simulink model "mpptmodel_newtest"  (Simulink 10.0)
settings: Solver=ode45  StartTime=0.0  StopTime=20  FixedStep=1e-8  RelTol=1e-3  EnableMultiTasking=on
libraries: powerlib x13, simulink x3
settings Model: Creator=Ranjith  LastModifiedBy=bhisma
settings DataIOCC: LimitDataPoints=on  SignalLoggingSaveFormat=ModelDataLogs
settings OptimizationCC: ExpressionDepthLimit=2147483647
settings DebuggingCC: SolverPrmCheckMsg=warning  MultiTaskRateTransMsg=warning  FcnCallInpInsideContextMsg=warning  StateNameClashWarn=warning
settings GRTTargetCC: GeneratePreprocessorConditionals=Disable all  CombineOutputUpdateFcns=on  GRTInterface=off
settings ConfigComp: CovExternalEMLEnable=off
settings SimscapeCC: SimscapeNormalizeSystem=off

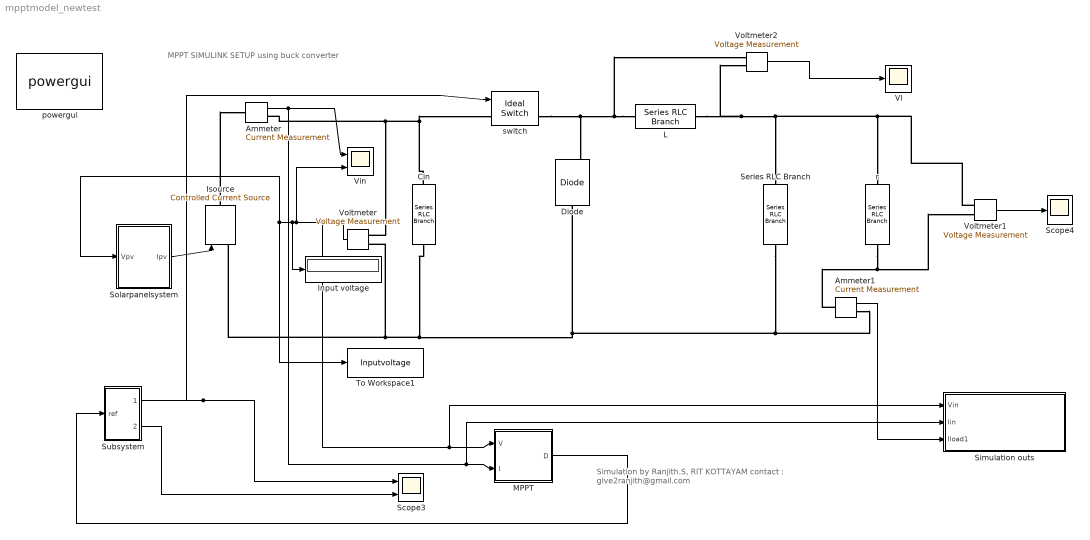
== system mpptmodel_newtest ==
  note: MPPT SIMULINK SETUP using buck converter
  note: Simulation by Ranjith.S, RIT KOTTAYAM
      |                          contact : give2ranjith@gmail.com
  Ammeter : powerlib/Measurements/Current Measurement  PhasorSimulation=off  OutputType=Complex  PSBequivalent=0
      settings: SourceProductName=Simscape Electrical
  Ammeter1 : powerlib/Measurements/Current Measurement  PhasorSimulation=off  OutputType=Complex  PSBequivalent=0
      settings: SourceProductName=Simscape Electrical
  Cin : powerlib/Elements/Series RLC Branch  LConnTagsString=__new0  RConnTagsString=__new0  BranchType=C  Resistance=0.03  Inductance=1e-3  SetiL0=off  InitialCurrent=0  Capacitance=2000e-6  Setx0=off  InitialVoltage=0  Measurements=None
      settings: SourceProductName=Simscape Electrical
  Diode : powerlib/Power Electronics/Diode  Ron=0.001  Lon=0  Vf=0.8  IC=0  UseSnubber=off  Rs=500  Cs=250e-9  Measurements=on
      settings: SourceProductName=Simscape Electrical
  Input voltage : Display
  Isource : powerlib/Electrical Sources/Controlled Current Source  Initialize=on  Source_Type=AC  Amplitude=0  Phase=0  Frequency=0  Measurements=None
      settings: SourceProductName=Simscape Electrical
  L : powerlib/Elements/Series RLC Branch  LConnTagsString=__new0  RConnTagsString=__new0  BranchType=L  Resistance=0.2e-3  Inductance=66e-6  SetiL0=off  InitialCurrent=0  Capacitance=1e-6  Setx0=off  InitialVoltage=0  Measurements=None
      settings: SourceProductName=Simscape Electrical
  MPPT : Subsystem
  Scope3 : Scope  NumInputPorts=2
  Scope4 : Scope
  Series RLC Branch : powerlib/Elements/Series RLC Branch  LConnTagsString=__new0  RConnTagsString=__new0  BranchType=RC  Resistance=0.0003  Inductance=1e-3  SetiL0=off  InitialCurrent=0  Capacitance=75e-6  Setx0=off  InitialVoltage=0  Measurements=None
      settings: SourceProductName=Simscape Electrical
  Simulation outs : Subsystem
  Solarpanelsystem : Subsystem
  Subsystem : Subsystem
  To Workspace1 : ToWorkspace  VariableName=Inputvoltage  SaveFormat=Timeseries  SampleTime=-1
  Vin : Scope  NumInputPorts=2
  Vl : Scope
  Voltmeter : powerlib/Measurements/Voltage Measurement  PhasorSimulation=off  OutputType=Complex  PSBequivalent=0
      settings: SourceProductName=Simscape Electrical
  Voltmeter1 : powerlib/Measurements/Voltage Measurement  PhasorSimulation=off  OutputType=Complex  PSBequivalent=0
      settings: SourceProductName=Simscape Electrical
  Voltmeter2 : powerlib/Measurements/Voltage Measurement  PhasorSimulation=off  OutputType=Complex  PSBequivalent=0
      settings: SourceProductName=Simscape Electrical
  powergui : powerlib/powergui  Priority=1  SimulationMode=Discrete  SolverType=Tustin  SampleTime=50e-6  frequency=60  SPID=on  DisableSnubberDevices=off  DisableRonSwitches=off  DisableVfSwitches=off  SwTol=0  Interpol=off  DisplayEquations=off  FunctionMessages=off  frequencyindice=0  Pbase=100e6  ErrMax=1e-4  Iterations=50  UnitsV=kV  UnitsW=MW  echomessages=off  HookPort=off  EnableUseOfTLC=off  x0status=blocks  RestoreLinks=warning  ResistiveCurrentMeasurement=off  Ylog=off  Xlog=on  ShowGrid=off  save=off  variable=ZData  ZoomFFT=off  StartTime=0.0  cycles=1  DisplayStyle=1  FreqAxis=off  MaxFrequency=1000  frequencyindicesteady=1  display=off  methode=off
      settings: SourceProductName=Simscape Electrical
  r : powerlib/Elements/Series RLC Branch  LConnTagsString=__new0  RConnTagsString=__new0  BranchType=R  Resistance=6  Inductance=1e-3  SetiL0=off  InitialCurrent=0  Capacitance=1e-6  Setx0=off  InitialVoltage=0  Measurements=None
      settings: SourceProductName=Simscape Electrical
  switch : powerlib/Power Electronics/Ideal Switch  Ron=0.001  Lon=0  IC=0  Rs=1e5  Cs=inf  Measurements=on
      settings: SourceProductName=Simscape Electrical
  wires:
  Voltmeter2/1 -> Vl/1
  Ammeter1/1 -> Simulation outs/3(Iload1)
  Voltmeter1/1 -> Scope4/1
  Ammeter/1 -> Vin/1, MPPT/2(I), Simulation outs/2(Iin)
  Voltmeter/1 -> Vin/2, Input voltage/1, Solarpanelsystem/1(Vpv), To Workspace1/1, MPPT/1(V), Simulation outs/1(Vin)
  Solarpanelsystem/1(Ipv) -> Isource/1
  Subsystem/1(pulse) -> Scope3/1, switch/1
  Subsystem/2(ramp) -> Scope3/2
  MPPT/1(D) -> Subsystem/1(ref)
  connections:
  r/RConn1 -- Ammeter1/LConn1 -- Voltmeter1/LConn2
  L/RConn1 -- r/LConn1 -- Voltmeter1/LConn1 -- Series RLC Branch/LConn1 -- Voltmeter2/LConn2
  L/LConn1 -- switch/RConn1 -- Diode/RConn1 -- Voltmeter2/LConn1
  Voltmeter/LConn2 -- Isource/LConn1 -- Diode/LConn1 -- Series RLC Branch/RConn1 -- Ammeter1/RConn1 -- Cin/RConn1
  Voltmeter/LConn1 -- Cin/LConn1 -- switch/LConn1 -- Ammeter/RConn1
  Isource/RConn1 -- Ammeter/LConn1

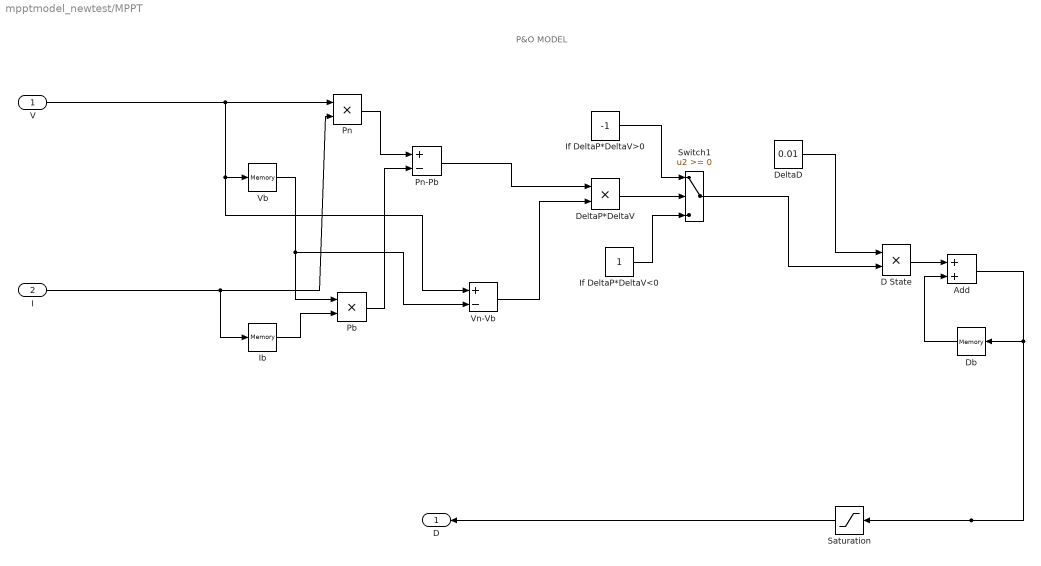
== system mpptmodel_newtest/MPPT ==
  note: P&O MODEL
  V : Inport
  I : Inport  Port=2
  Add : Sum
  D State : Product  RndMeth=Zero
  Db : Memory  InheritSampleTime=on  LinearizeAsDelay=on
  DeltaD : Constant  Value=0.01
  DeltaP*DeltaV : Product  RndMeth=Zero
  Ib : Memory  InheritSampleTime=on  LinearizeAsDelay=on
  If DeltaP*DeltaV<0 : Constant
  If DeltaP*DeltaV>0 : Constant  Value=-1
  Pb : Product  RndMeth=Zero
  Pn : Product  RndMeth=Zero
  Pn-Pb : Sum  Inputs=+-
  Saturation : Saturate  UpperLimit=.9  LowerLimit=.1
  Switch1 : Switch
  Vb : Memory  InheritSampleTime=on  LinearizeAsDelay=on
  Vn-Vb : Sum  Inputs=+-
  D : Outport
  wires:
  V/1 -> Pn/1, Vb/1, Vn-Vb/1
  I/1 -> Ib/1, Pn/2
  Ib/1 -> Pb/2
  Vb/1 -> Pb/1, Vn-Vb/2
  Pn/1 -> Pn-Pb/1
  Pb/1 -> Pn-Pb/2
  D State/1 -> Add/1
  Add/1 -> Db/1, Saturation/1
  Db/1 -> Add/2
  Pn-Pb/1 -> DeltaP*DeltaV/1
  Vn-Vb/1 -> DeltaP*DeltaV/2
  DeltaP*DeltaV/1 -> Switch1/2
  If DeltaP*DeltaV>0/1 -> Switch1/1
  If DeltaP*DeltaV<0/1 -> Switch1/3
  Switch1/1 -> D State/2
  DeltaD/1 -> D State/1
  Saturation/1 -> D/1

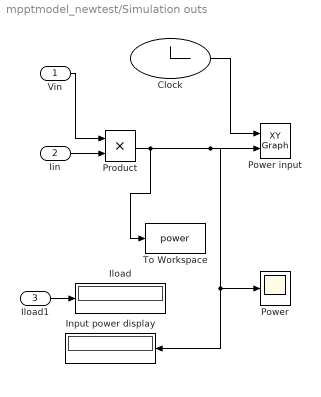
== system mpptmodel_newtest/Simulation outs ==
  Vin : Inport
  Iin : Inport  Port=2
  Iload1 : Inport  Port=3
  Clock : Clock
  Iload : Display
  Input power display : Display
  Power : Scope
  Power input : simulink/Sinks/XY Graph  xmin=0  xmax=0.1  ymin=0  ymax=100  st=-1
  Product : Product  RndMeth=Zero
  To Workspace : ToWorkspace  VariableName=power  SaveFormat=Timeseries  SampleTime=-1
  wires:
  Product/1 -> To Workspace/1, Input power display/1, Power/1, Power input/2
  Clock/1 -> Power input/1
  Vin/1 -> Product/1
  Iin/1 -> Product/2
  Iload1/1 -> Iload/1

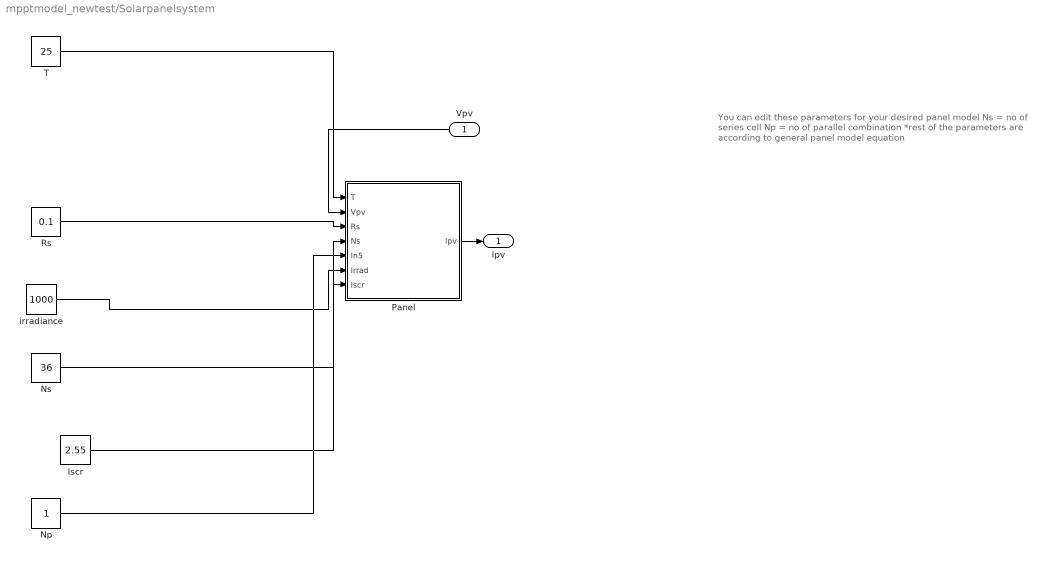
== system mpptmodel_newtest/Solarpanelsystem ==
  note: You can edit these parameters for your desired panel model
      |
      | Ns = no of series cell
      | Np = no of parallel combination
      |
      | *rest of the parameters are according to general panel model equation
  Vpv : Inport
  Iscr : Constant  Value=2.55
  Np : Constant
  Ns : Constant  Value=36
  Panel : Subsystem
  Rs : Constant  Value=0.1
  T : Constant  Value=25
  irradiance : Constant  Value=1000
  Ipv : Outport
  wires:
  Rs/1 -> Panel/3(Rs)
  Np/1 -> Panel/5(In5)
  T/1 -> Panel/1(T)
  Ns/1 -> Panel/4(Ns)
  Iscr/1 -> Panel/7(Iscr)
  Panel/1(Ipv) -> Ipv/1
  Vpv/1 -> Panel/2(Vpv)
  irradiance/1 -> Panel/6(Irrad)

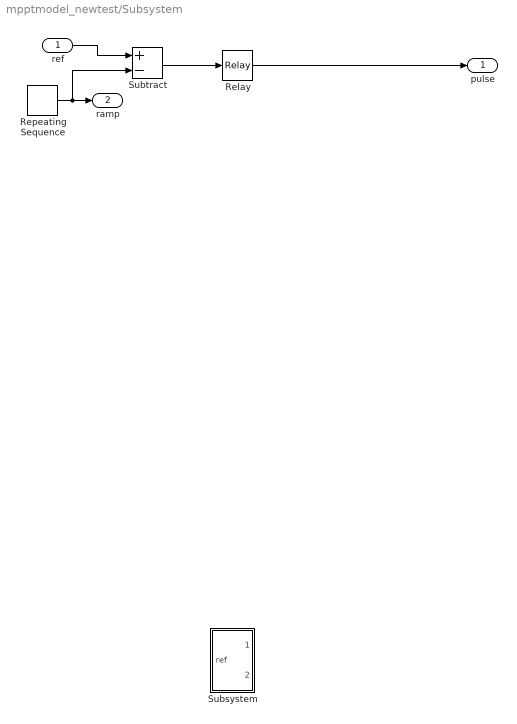
== system mpptmodel_newtest/Subsystem ==
  ref : Inport
  Relay : Relay
  Repeating Sequence : simulink/Sources/Repeating Sequence  rep_seq_t=[0 0.02e-3 0.02e-3]  rep_seq_y=[0 1 0]
  Subsystem : Subsystem
  Subtract : Sum  Inputs=+-
  pulse : Outport
  ramp : Outport  Port=2
  wires:
  Repeating Sequence/1 -> ramp/1, Subtract/2
  ref/1 -> Subtract/1
  Relay/1 -> pulse/1
  Subtract/1 -> Relay/1

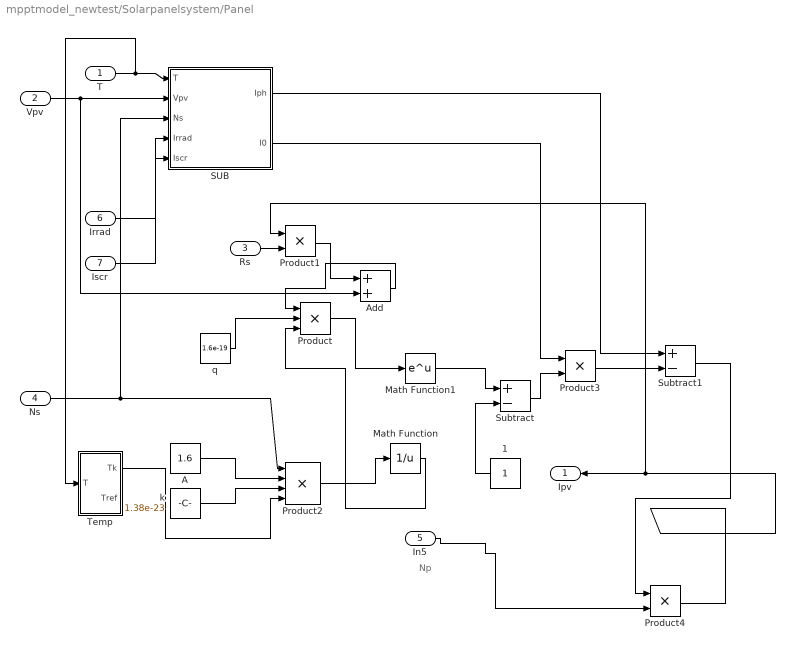
== system mpptmodel_newtest/Solarpanelsystem/Panel ==
  note: Np
  T : Inport
  Vpv : Inport  Port=2
  Rs : Inport  Port=3
  Ns : Inport  Port=4
  In5 : Inport  Port=5
  Irrad : Inport  Port=6
  Iscr : Inport  Port=7
  1 : Constant
  A : Constant  Value=1.6
  Add : Sum
  Math Function : Math  Operator=reciprocal  SaturateOnIntegerOverflow=on
  Math Function1 : Math  SaturateOnIntegerOverflow=on
  Product : Product  Inputs=3  RndMeth=Zero
  Product1 : Product  RndMeth=Zero
  Product2 : Product  Inputs=4  RndMeth=Zero
  Product3 : Product  RndMeth=Zero
  Product4 : Product  RndMeth=Zero
  SUB : Subsystem
  Subtract : Sum  Inputs=+-
  Subtract1 : Sum  Inputs=+-
  Temp : Subsystem
  k : Constant  Value=1.38e-23
  q : Constant  Value=1.6e-19
  Ipv : Outport
  wires:
  T/1 -> SUB/1(T), Temp/1(T)
  Vpv/1 -> SUB/2(Vpv), Add/2
  q/1 -> Product/2
  Product1/1 -> Add/1
  Add/1 -> Product/1
  k/1 -> Product2/3
  A/1 -> Product2/2
  Ns/1 -> Product2/1, SUB/3(Ns)
  Product2/1 -> Math Function/1
  Math Function/1 -> Product/3
  Product/1 -> Math Function1/1
  Math Function1/1 -> Subtract/1
  1/1 -> Subtract/2
  SUB/1(Iph) -> Subtract1/1
  SUB/2(I0) -> Product3/1
  Subtract/1 -> Product3/2
  Product3/1 -> Subtract1/2
  Subtract1/1 -> Product4/1
  Rs/1 -> Product1/2
  In5/1 -> Product4/2
  Irrad/1 -> SUB/4(Irrad)
  Iscr/1 -> SUB/5(Iscr)
  Temp/1(Tk) -> Product2/4
  Product4/1 -> Ipv/1, Product1/1

== system mpptmodel_newtest/Subsystem/Subsystem ==
  ref : Inport
  Relay : Relay
  Repeating Sequence : simulink/Sources/Repeating Sequence  rep_seq_t=[0:0.001e-3:0.02e-3]  rep_seq_y=[0:0.1:2]
  Subtract : Sum  Inputs=+-
  pulse : Outport
  ramp : Outport  Port=2
  wires:
  Relay/1 -> pulse/1
  ref/1 -> Subtract/1
  Subtract/1 -> Relay/1
  Repeating Sequence/1 -> ramp/1, Subtract/2

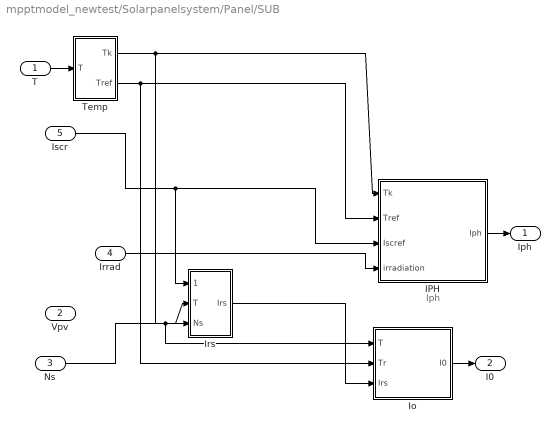
== system mpptmodel_newtest/Solarpanelsystem/Panel/SUB ==
  note: Iph
  T : Inport
  Vpv : Inport  Port=2
  Ns : Inport  Port=3
  Irrad : Inport  Port=4
  Iscr : Inport  Port=5
  IPH : Subsystem
  Io : Subsystem
  Irs : Subsystem
  Temp : Subsystem
  Iph : Outport
  I0 : Outport  Port=2
  wires:
  Temp/1(Tk) -> IPH/1(Tk), Irs/2(T), Io/1(T)
  Temp/2(Tref) -> IPH/2(Tref), Io/2(Tr)
  Irrad/1 -> IPH/4(irradiation)
  Irs/1(Irs) -> Io/3(Irs)
  T/1 -> Temp/1(T)
  IPH/1(Iph) -> Iph/1
  Io/1(I0) -> I0/1
  Ns/1 -> Irs/3(Ns)
  Iscr/1 -> IPH/3(Iscref), Irs/1(Iscr)

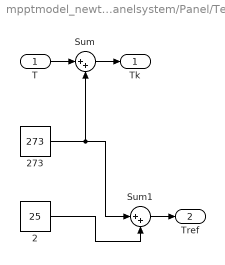
== system mpptmodel_newtest/Solarpanelsystem/Panel/Temp ==
  T : Inport
  2 : Constant  Value=25
  273 : Constant  Value=273
  Sum : Sum  Inputs=|++
  Sum1 : Sum  Inputs=|++
  Tk : Outport
  Tref : Outport  Port=2
  wires:
  273/1 -> Sum/2, Sum1/1
  2/1 -> Sum1/2
  T/1 -> Sum/1
  Sum/1 -> Tk/1
  Sum1/1 -> Tref/1

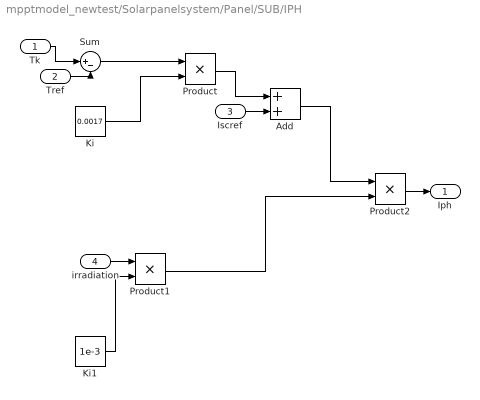
== system mpptmodel_newtest/Solarpanelsystem/Panel/SUB/IPH ==
  Tk : Inport
  Tref : Inport  Port=2
  Iscref : Inport  Port=3
  irradiation : Inport  Port=4
  Add : Sum
  Ki : Constant  Value=0.0017
  Ki1 : Constant  Value=1e-3
  Product : Product  RndMeth=Zero
  Product1 : Product  RndMeth=Zero
  Product2 : Product  RndMeth=Zero
  Sum : Sum  Inputs=|+-
  Iph : Outport
  wires:
  Sum/1 -> Product/1
  Ki/1 -> Product/2
  Product/1 -> Add/1
  Ki1/1 -> Product1/2
  Product1/1 -> Product2/2
  Add/1 -> Product2/1
  Tk/1 -> Sum/1
  Tref/1 -> Sum/2
  Iscref/1 -> Add/2
  Product2/1 -> Iph/1
  irradiation/1 -> Product1/1

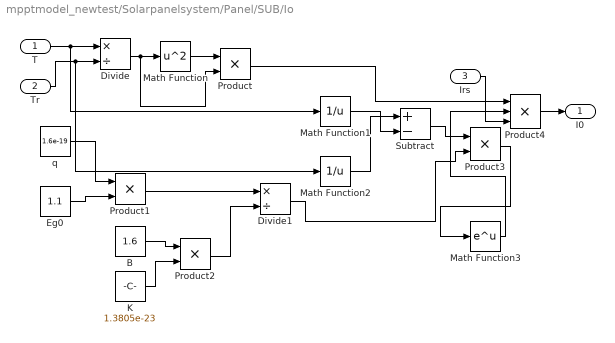
== system mpptmodel_newtest/Solarpanelsystem/Panel/SUB/Io ==
  T : Inport
  Tr : Inport  Port=2
  Irs : Inport  Port=3
  B : Constant  Value=1.6
  Divide : Product  Inputs=*/
  Divide1 : Product  Inputs=*/
  Eg0 : Constant  Value=1.1
  K : Constant  Value=1.3805e-23
  Math Function : Math  Operator=square  SaturateOnIntegerOverflow=on
  Math Function1 : Math  Operator=reciprocal  SaturateOnIntegerOverflow=on
  Math Function2 : Math  Operator=reciprocal  SaturateOnIntegerOverflow=on
  Math Function3 : Math  SaturateOnIntegerOverflow=on
  Product{,1..3} (4 alike) : Product  RndMeth=Zero
  Product4 : Product  Inputs=3  RndMeth=Zero
  Subtract : Sum  Inputs=+-
  q : Constant  Value=1.6e-19
  I0 : Outport
  wires:
  Divide/1 -> Math Function/1, Product/2
  Math Function/1 -> Product/1
  q/1 -> Product1/1
  Eg0/1 -> Product1/2
  B/1 -> Product2/1
  K/1 -> Product2/2
  Product1/1 -> Divide1/1
  Product2/1 -> Divide1/2
  Math Function2/1 -> Subtract/1
  Math Function1/1 -> Subtract/2
  Subtract/1 -> Product3/1
  Divide1/1 -> Product3/2
  Product3/1 -> Math Function3/1
  Math Function3/1 -> Product4/2
  Product/1 -> Product4/1
  T/1 -> Divide/1, Math Function1/1
  Tr/1 -> Divide/2, Math Function2/1
  Product4/1 -> I0/1
  Irs/1 -> Product4/3

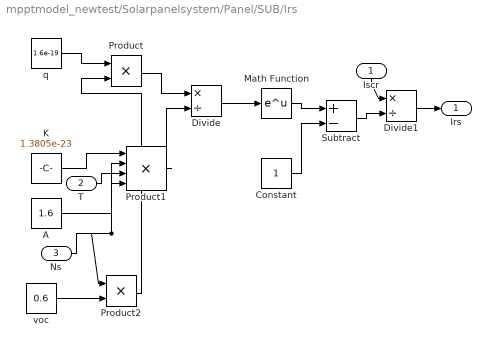
== system mpptmodel_newtest/Solarpanelsystem/Panel/SUB/Irs ==
  Iscr : Inport
  T : Inport  Port=2
  Ns : Inport  Port=3
  A : Constant  Value=1.6
  Constant : Constant
  Divide : Product  Inputs=*/
  Divide1 : Product  Inputs=*/
  K : Constant  Value=1.3805e-23
  Math Function : Math  SaturateOnIntegerOverflow=on
  Product : Product  RndMeth=Zero
  Product1 : Product  Inputs=4  RndMeth=Zero
  Product2 : Product  RndMeth=Zero
  Subtract : Sum  Inputs=+-
  q : Constant  Value=1.6e-19
  voc : Constant  Value=0.6
  Irs : Outport
  wires:
  q/1 -> Product/1
  K/1 -> Product1/1
  A/1 -> Product1/2
  Product/1 -> Divide/1
  Product1/1 -> Divide/2
  Divide/1 -> Math Function/1
  Math Function/1 -> Subtract/1
  Constant/1 -> Subtract/2
  Subtract/1 -> Divide1/2
  Iscr/1 -> Divide1/1
  T/1 -> Product1/3
  Divide1/1 -> Irs/1
  Ns/1 -> Product1/4, Product2/1
  voc/1 -> Product2/2
  Product2/1 -> Product/2

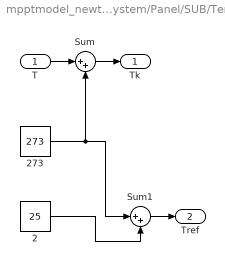
== system mpptmodel_newtest/Solarpanelsystem/Panel/SUB/Temp ==
  T : Inport
  2 : Constant  Value=25
  273 : Constant  Value=273
  Sum : Sum  Inputs=|++
  Sum1 : Sum  Inputs=|++
  Tk : Outport
  Tref : Outport  Port=2
  wires:
  273/1 -> Sum/2, Sum1/1
  2/1 -> Sum1/2
  T/1 -> Sum/1
  Sum/1 -> Tk/1
  Sum1/1 -> Tref/1
